simulink model "MAC_ADC"  (R2021a)
settings: Solver=VariableStepAuto  StartTime=0.0  StopTime=1  RelTol=1e-3
values from neighbouring files (symbols this model uses):
  C2 = 2*nb_MAC*minimum_cap    [MAC_ADC_main.m]
  Cf = minimum_cap    [MAC_ADC_main.m]
  clk_freq = 2.1*(nb_cycles_per_sample/(nb_MAC))*sine_frequency_rad    (= 5742.32871594)    [MAC_ADC_main.m]
  clk_period = 1/clk_freq    (= 0.000174145377158)    [MAC_ADC_main.m]
  comparator_high_offset = 0.2*10e-4    (= 0.0002)    [MAC_ADC_main.m]
  comparator_low_offset = -.1*10e-4    (= -0.0001)    [MAC_ADC_main.m]
  comparator_noise_on = non_idealities_on    (= 0)    [MAC_ADC_main.m]
  comparator_noise_rms = 1*k*T* 2/3 / minimum_cap    [MAC_ADC_main.m]
  comparator_offset_on = non_idealities_on    (= 0)    [MAC_ADC_main.m]
  input_BW = 256    [MAC_ADC_main.m]
  k = 1.38064852e-23    [MAC_ADC_main.m]
  leak_current = 2e-15    [MAC_ADC_main.m]
  LNA_bandwidth = 3*input_BW    (= 768)    [MAC_ADC_main.m]
  LNA_gain = 100    [MAC_ADC_main.m]
  LNA_input_referred_noise = min([LNA_input_referred_noise_1,LNA_input_referred_noise_2,LNA_input_referred_noise_3])    [MAC_ADC_main.m]
  LNA_noise_on = non_idealities_on    (= 0)    [MAC_ADC_main.m]
  LNA_SR = I_LNA/(minimum_cap)    [MAC_ADC_main.m]
  MM_attenuation_coeff = C2/(C1+C2)    [MAC_ADC_main.m]
  MM_incomplete_transfer_coeff = C1/(C1+C2)    [MAC_ADC_main.m]
  MM_sampling_noise = ((k*T * C1 / (C1+C2)^2) + (k*T*(C1*C2/(C1+C2))/C2^2))^1/2    [MAC_ADC_main.m]
  nb_cycles_per_sample = number_of_bits + 4 + nb_MAC    (= 34)    [MAC_ADC_main.m]
  nb_MAC = 20    [MAC_ADC_main.m]
  noise_seed = 1    [MAC_ADC_main.m]
  number_of_bits = 10    [MAC_ADC_main.m]
  sampling_gain = Cs/Cf    [MAC_ADC_main.m]
  switch_noise_on = non_idealities_on    (= 0)    [MAC_ADC_main.m]
  switching_noise = k*T/Cf    [MAC_ADC_main.m]
  T = 293    [MAC_ADC_main.m]
  Vref = 2    [MAC_ADC_main.m]
  ZOH_delta = 0*Vref/(2^number_of_bits)    (= 0)    [MAC_ADC_main.m]
libraries: dspsigops x2, simulink x2, simulink_extras x2, spsFirstOrderFilterLib x1, dspsrcs4 x1, dspswit3 x1
settings Model: SnapshotInterval=1  Creator=mac  LastModifiedBy=mac
settings SolverCC: AlgebraicLoopSolver=TrustRegion
settings DataIOCC: SaveFormat=Structure  OutputOption=SpecifiedOutputTimes  OutputTimes=[0:(nb_cycles_per_sample)*clk_period:nb_cycles_per_sample*clk_period*(nb_samples+1)]
settings DebuggingCC: SFMachineParentedDataDiag=warning  UnderSpecifiedDimensionMsg=warning

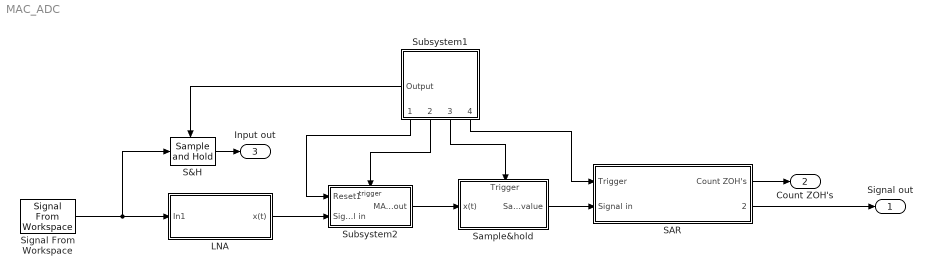
== system MAC_ADC ==
  LNA : Subsystem
      mask Display: text(.5, .5, 'LNA', 'horizontalAlignment', 'center', 'verticalAlignment', 'middle')
  S&H : dspsigops/Sample and Hold  trig=Rising edge  initCond=0  latchinput=off
  SAR : Subsystem
      mask Display: text(.5, .5, 'ZOH SAR', 'horizontalAlignment', 'center', 'verticalAlignment', 'middle')
  Sample&hold : Subsystem
      settings: PortSchema="{\"entries\":[{\"content\":{\"sides\":[{\"content\":{\"connectorIds\":[\"In1\"]},\"type\":\"ConnectorPlacement.EquallySpacedRectSide\",\"uuid\":\"7dc7a4da-613e-4b0b-8b13-7686a16d7398\"},{\"content\":{\"connectorIds\":[\"Out1\"],\"side\":\"RIGHT\"},\"type\":\"ConnectorPlacement.EquallySpacedRectSide\",\"uuid\":\"45e05abc-e512-455b-8082-6639e5b5b38c\"},{\"content\":{\"connectorIds\":[\"In2\"],\"side\":\"TOP\"},\"type\":\"ConnectorPlacement.EquallySpacedRectSide\",\"uuid\":\"b599ec83-17db-48a3-a9e2-86d99bd6436c\"},{\"content\":{\"connectorIds\":[],\"side\":\"HIDDEN\"},\"type\":\"ConnectorPlacement.EquallySpacedRectSide\",\"uuid\":\"38635b0c-9992-4d58-9e3d-95a04571faab\"}]},\"type\":\"ConnectorPlacement.EquallySpacedConnector\",\"uuid\":\"ba0d73a9-648c-4aab-96ad-c6572107f92b\"}],\"packageUris\":[\"http://schema.mathworks.com/mf0/Connector/R2020b\"],\"version\":\"1.0\"}"
      mask Display: text(.5, .5, 'Sample & hold', 'horizontalAlignment', 'center', 'verticalAlignment', 'middle')
  Signal From Workspace : dspsrcs4/Signal From Workspace  X=ADC_input  Ts=1/input_BW  nsamps=1  OutputAfterFinalValue=Setting to zero  ignoreOrWarnInputAndFrameLengths=off  OutputFrames=off
  Subsystem1 : Subsystem
      settings: PortSchema="{\"entries\":[{\"content\":{\"sides\":[{\"content\":{\"connectorIds\":[]},\"type\":\"ConnectorPlacement.EquallySpacedRectSide\",\"uuid\":\"08b362f4-e51c-4c48-9795-383a666f9ced\"},{\"content\":{\"connectorIds\":[\"Out1\",\"Out2\",\"Out3\",\"Out4\"],\"side\":\"RIGHT\"},\"type\":\"ConnectorPlacement.EquallySpacedRectSide\",\"uuid\":\"c1079507-a800-4a5f-bf86-70ea93d83d34\"},{\"content\":{\"connectorIds\":[\"Out5\"],\"side\":\"TOP\"},\"type\":\"ConnectorPlacement.EquallySpacedRectSide\",\"uuid\":\"869febc6-8a73-4083-9381-541b01b45ea7\"},{\"content\":{\"connectorIds\":[],\"side\":\"HIDDEN\"},\"type\":\"ConnectorPlacement.EquallySpacedRectSide\",\"uuid\":\"c096a564-5078-4383-9edd-02cc8c4f8a61\"}]},\"type\":\"ConnectorPlacement.EquallySpacedConnector\",\"uuid\":\"f254d905-503c-4801-8edf-b87de2253b64\"}],\"packageUris\":[\"http://schema.mathworks.com/mf0/Connector/R2020b\"],\"version\":\"1.0\"}"
      mask Display: text(.5, .5, 'Clocking block', 'horizontalAlignment', 'center', 'verticalAlignment', 'middle')
  Subsystem2 : Subsystem
      mask Display: text(.5, .5, 'MAC', 'horizontalAlignment', 'center', 'verticalAlignment', 'middle')
  Signal out : Outport
  Count ZOH's : Outport  Port=2
  Input out : Outport  Port=3
  wires:
  S&H/1 -> Input out/1
  Sample&hold/1(Sampled value) -> SAR/2(Signal in)
  SAR/1(Count ZOH's) -> Count ZOH's/1
  SAR/2(" ") -> Signal out/1
  Subsystem1/4(Output2) -> SAR/1(Trigger)
  Subsystem1/3(Output3) -> Sample&hold/2(Trigger)
  Subsystem1/2(MAC trigger) -> Subsystem2/Trigger
  Subsystem1/1(Output1) -> Subsystem2/1(Reset1)
  Subsystem2/1(MAC_out) -> Sample&hold/1(x(t))
  LNA/1(x(t)) -> Subsystem2/2(Signal in)
  Signal From Workspace/1 -> S&H/1, LNA/1(In1)
  Subsystem1/5(Output) -> S&H/Trigger

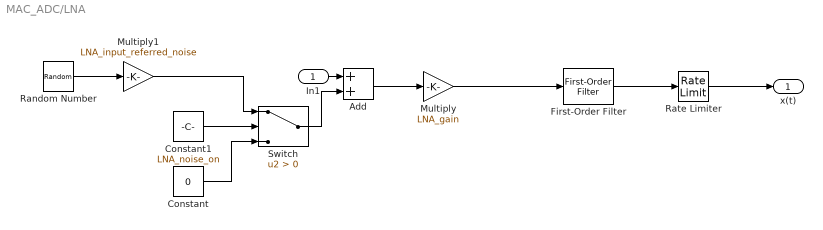
== system MAC_ADC/LNA ==
  In1 : Inport
  Add : Sum
  Constant : Constant  Value=0
  Constant1 : Constant  Value=LNA_noise_on
  First-Order Filter : spsFirstOrderFilterLib/First-Order Filter  FilterType=Lowpass  Tc=1/(LNA_bandwidth*2*pi)  Ts=0  Initialize=off  Vac_Init=[0, 0, 60]  Vdc_Init=0  PlotResponse=off  FreqRange="[0,  200,  1]"
  Multiply : Gain  Gain=LNA_gain
  Multiply1 : Gain  Gain=LNA_input_referred_noise
  Random Number : RandomNumber  Seed=noise_seed+8  SampleTime=clk_period*(number_of_bits+1)
  Rate Limiter : RateLimiter  RisingSlewLimit=LNA_SR  FallingSlewLimit=-LNA_SR  SampleTimeMode=inherited
  Switch : Switch  Criteria=u2 > Threshold
  x(t) : Outport
  wires:
  In1/1 -> Add/1
  Random Number/1 -> Multiply1/1
  Add/1 -> Multiply/1
  Multiply1/1 -> Switch/1
  Constant/1 -> Switch/3
  Constant1/1 -> Switch/2
  Switch/1 -> Add/2
  Multiply/1 -> First-Order Filter/1
  Rate Limiter/1 -> x(t)/1
  First-Order Filter/1 -> Rate Limiter/1

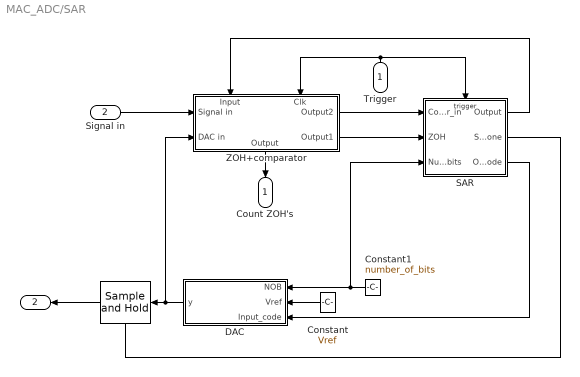
== system MAC_ADC/SAR ==
  Trigger : Inport
  Signal in : Inport  Port=2
  "           " : dspsigops/Sample and Hold  trig=Rising edge  initCond=0  latchinput=off
  Constant : Constant  Value=Vref
  Constant1 : Constant  Value=number_of_bits
  DAC : Subsystem  TreatAsAtomicUnit=on
      mask Display: text(.5, .5, 'DAC', 'horizontalAlignment', 'center', 'verticalAlignment', 'middle')
  SAR : Subsystem  TreatAsAtomicUnit=on
      mask Display: text(.5, .5, 'SAR', 'horizontalAlignment', 'center', 'verticalAlignment', 'middle')
  ZOH+comparator : Subsystem
      settings: PortSchema="{\"entries\":[{\"content\":{\"sides\":[{\"content\":{\"connectorIds\":[\"In1\",\"In2\"]},\"type\":\"ConnectorPlacement.EquallySpacedRectSide\",\"uuid\":\"7512c97b-848f-4506-b4e4-df4323ddef76\"},{\"content\":{\"connectorIds\":[\"Out1\",\"Out2\"],\"side\":\"RIGHT\"},\"type\":\"ConnectorPlacement.EquallySpacedRectSide\",\"uuid\":\"173ab639-376f-4392-8113-9f10a64ef5ba\"},{\"content\":{\"connectorIds\":[\"In3\",\"In4\"],\"side\":\"TOP\"},\"type\":\"ConnectorPlacement.EquallySpacedRectSide\",\"uuid\":\"b167df5d-9d76-4988-887c-42eca149e1c8\"},{\"content\":{\"connectorIds\":[\"Out3\"],\"side\":\"BOTTOM\"},\"type\":\"ConnectorPlacement.EquallySpacedRectSide\",\"uuid\":\"853aabd3-db33-416b-be96-d4661842c69c\"},{\"content\":{\"connectorIds\":[],\"side\":\"HIDDEN\"},\"type\":\"ConnectorPlacement.EquallySpacedRectSide\",\"uuid\":\"e2358589-1082-44c0-a092-f45782973cce\"}]},\"type\":\"ConnectorPlacement.EquallySpacedConnector\",\"uuid\":\"7d04fd09-a295-4450-8277-4727e6a38cb5\"}],\"packageUris\":[\"http://schema.mathworks.com/mf0/Connector/R2020b\"],\"version\":\"1.0\"}"
      mask Display: text(.5, .5, 'Comparator', 'horizontalAlignment', 'center', 'verticalAlignment', 'middle')
  Count ZOH's : Outport
  " " : Outport  Port=2
  wires:
  SAR/2(SAR_done) -> "           "/Trigger
  ZOH+comparator/3(Output) -> Count ZOH's/1
  SAR/3(Output_code) -> DAC/3(Input_code)
  "           "/1 -> " "/1
  Constant/1 -> DAC/2(Vref)
  ZOH+comparator/1(Output2) -> SAR/1(Comparator_in)
  Signal in/1 -> ZOH+comparator/1(Signal in)
  Constant1/1 -> SAR/3(Number of bits), DAC/1(NOB)
  DAC/1(y) -> ZOH+comparator/2(DAC in), "           "/1
  ZOH+comparator/2(Output1) -> SAR/2(ZOH)
  SAR/1(Output) -> ZOH+comparator/3(Input)
  Trigger/1 -> ZOH+comparator/4(Clk), SAR/Trigger

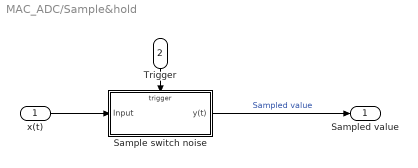
== system MAC_ADC/Sample&hold ==
  x(t) : Inport
  Trigger : Inport  Port=2
  Sample switch noise : Subsystem  TreatAsAtomicUnit=on
  Sampled value : Outport
  wires:
  Trigger/1 -> Sample switch noise/Trigger
  Sample switch noise/1(y(t)) -> Sampled value/1  "Sampled value"
  x(t)/1 -> Sample switch noise/1(Input)

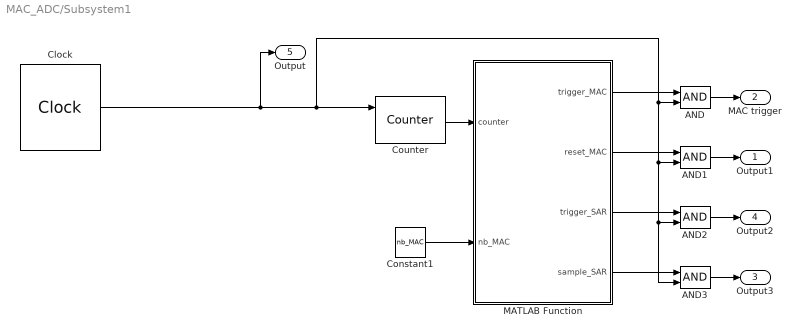
== system MAC_ADC/Subsystem1 ==
  AND{,1..3} (4 alike) : Logic  IconShape=distinctive  AllPortsSameDT=off  OutDataTypeStr=boolean
  Clock : simulink_extras/Flip Flops/Clock  period=clk_period
  Constant1 : Constant  Value=nb_MAC
  Counter : dspswit3/Counter  Direction=Up  CountEvent=Rising edge  CounterSize=User defined  MaxCount=nb_cycles_per_sample-1  InitialCount=0  Output=Count  HitValue=32  ResetInput=on  SamplesPerFrame=1  Ts=1  CntDtype=double  HitDtype=Logical
  MATLAB Function : MATLAB Function  TreatAsAtomicUnit=on
  Output1 : Outport
  MAC trigger : Outport  Port=2
  Output3 : Outport  Port=3
  Output2 : Outport  Port=4
  Output : Outport  Port=5
  wires:
  Clock/1 -> Output/1, Counter/1, AND2/2, AND3/2, AND1/2, AND/2
  Counter/1 -> MATLAB Function/1(counter)
  Constant1/1 -> MATLAB Function/2(nb_MAC)
  AND/1 -> MAC trigger/1
  AND1/1 -> Output1/1
  AND2/1 -> Output2/1
  AND3/1 -> Output3/1
  MATLAB Function/4(sample_SAR) -> AND3/1
  MATLAB Function/3(trigger_SAR) -> AND2/1
  MATLAB Function/2(reset_MAC) -> AND1/1
  MATLAB Function/1(trigger_MAC) -> AND/1

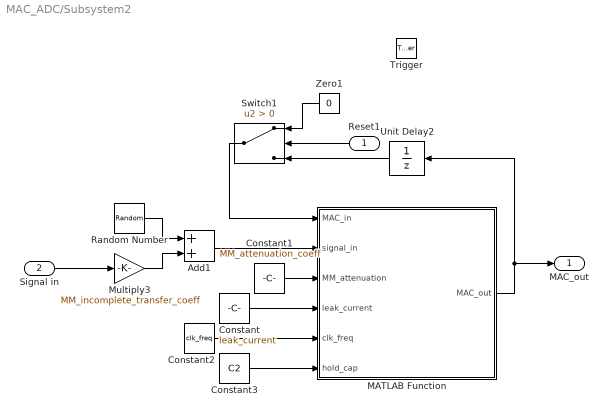
== system MAC_ADC/Subsystem2 ==
  Reset1 : Inport
  Signal in : Inport  Port=2
  Trigger : TriggerPort  VariantControl=Variant  PortDimensions=1
  Add1 : Sum
  Constant : Constant  Value=leak_current
  Constant1 : Constant  Value=MM_attenuation_coeff
  Constant2 : Constant  Value=clk_freq
  Constant3 : Constant  Value=C2
  MATLAB Function : MATLAB Function  TreatAsAtomicUnit=on
  Multiply3 : Gain  Gain=MM_incomplete_transfer_coeff
  Random Number : RandomNumber  Variance=MM_sampling_noise  Seed=noise_seed+2398
  Switch1 : Switch  Criteria=u2 > Threshold
  Unit Delay2 : UnitDelay  InitialCondition=1  SampleTime=-1  HasFrameUpgradeWarning=on
  Zero1 : Constant  Value=0  OutDataTypeStr=Inherit: Inherit via back propagation
  MAC_out : Outport
  wires:
  Zero1/1 -> Switch1/1
  Random Number/1 -> Add1/1
  MATLAB Function/1(MAC_out) -> Unit Delay2/1, MAC_out/1
  Reset1/1 -> Switch1/2
  Constant1/1 -> MATLAB Function/3(MM_attenuation)
  Constant2/1 -> MATLAB Function/5(clk_freq)
  Add1/1 -> MATLAB Function/2(signal_in)
  Signal in/1 -> Multiply3/1
  Multiply3/1 -> Add1/2
  Unit Delay2/1 -> Switch1/3
  Switch1/1 -> MATLAB Function/1(MAC_in)
  Constant/1 -> MATLAB Function/4(leak_current)
  Constant3/1 -> MATLAB Function/6(hold_cap)

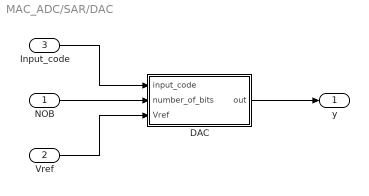
== system MAC_ADC/SAR/DAC ==
  NOB : Inport
  Vref : Inport  Port=2
  Input_code : Inport  Port=3
  DAC : MATLAB Function  TreatAsAtomicUnit=on
  y : Outport
  wires:
  NOB/1 -> DAC/2(number_of_bits)
  Vref/1 -> DAC/3(Vref)
  DAC/1(out) -> y/1
  Input_code/1 -> DAC/1(input_code)

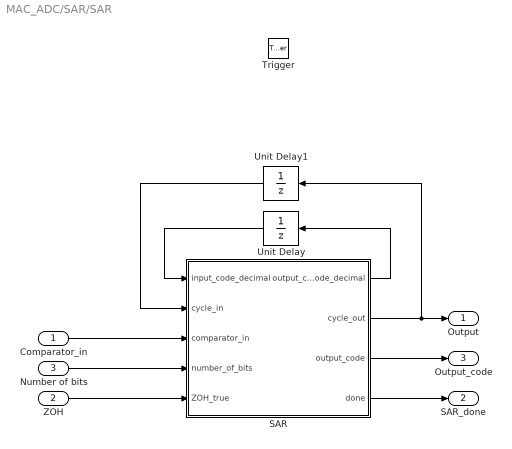
== system MAC_ADC/SAR/SAR ==
  Comparator_in : Inport  LatchByDelayingOutsideSignal=on
  ZOH : Inport  Port=2  LatchByDelayingOutsideSignal=on
  Number of bits : Inport  Port=3
  Trigger : TriggerPort  VariantControl=Variant
  SAR : MATLAB Function  TreatAsAtomicUnit=on
  Unit Delay : UnitDelay  SampleTime=-1  HasFrameUpgradeWarning=on
  Unit Delay1 : UnitDelay  SampleTime=-1  HasFrameUpgradeWarning=on
  Output : Outport
  SAR_done : Outport  Port=2  InitialOutput=0
  Output_code : Outport  Port=3  InitialOutput=zeros(number_of_bits, 1)
      settings: VarSizeSig=Yes
  wires:
  Number of bits/1 -> SAR/4(number_of_bits)
  Comparator_in/1 -> SAR/3(comparator_in)
  Unit Delay1/1 -> SAR/2(cycle_in)
  SAR/3(output_code) -> Output_code/1
  Unit Delay/1 -> SAR/1(input_code_decimal)
  SAR/1(output_code_decimal) -> Unit Delay/1
  SAR/4(done) -> SAR_done/1
  ZOH/1 -> SAR/5(ZOH_true)
  SAR/2(cycle_out) -> Output/1, Unit Delay1/1

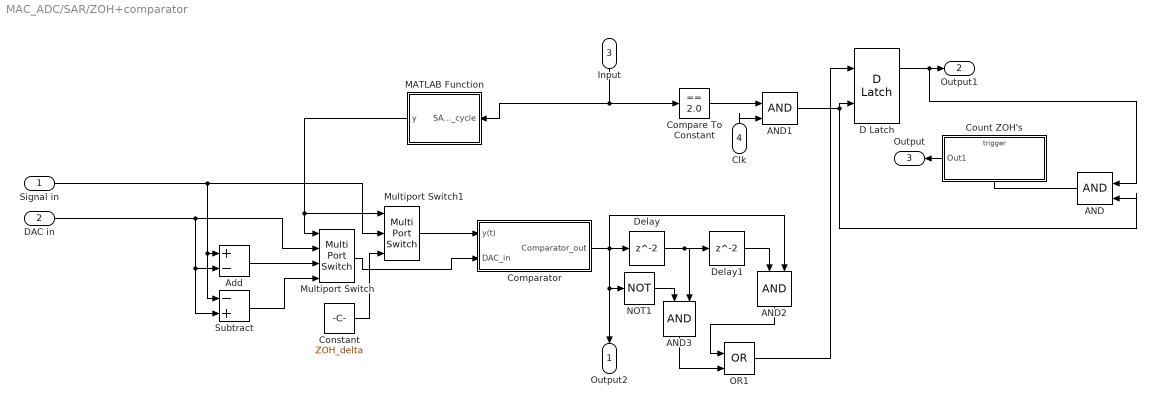
== system MAC_ADC/SAR/ZOH+comparator ==
  Signal in : Inport
  DAC in : Inport  Port=2
  Input : Inport  Port=3
  Clk : Inport  Port=4
  AND{,1..3} (4 alike) : Logic  IconShape=distinctive  AllPortsSameDT=off  OutDataTypeStr=boolean
  Add : Sum  Inputs=+-
  Comparator : Subsystem  TreatAsAtomicUnit=on
      mask Display: text(.5, .5, 'Comparator', 'horizontalAlignment', 'center', 'verticalAlignment', 'middle')
  Compare To Constant : simulink/Logic and Bit Operations/Compare To Constant  relop===  const=2.0  OutDataTypeStr=boolean
  Constant : Constant  Value=ZOH_delta
  Count ZOH's : Subsystem
  D Latch : simulink_extras/Flip Flops/D Latch
      settings: SourceProductBaseCode=SL
  Delay : Delay
  Delay1 : Delay
  MATLAB Function : MATLAB Function  TreatAsAtomicUnit=on
  Multiport Switch : MultiPortSwitch
  Multiport Switch1 : MultiPortSwitch  Inputs=2  DiagnosticForDefault=None
  NOT1 : Logic  Operator=NOT  IconShape=distinctive  AllPortsSameDT=off  OutDataTypeStr=boolean
  OR1 : Logic  Operator=OR  IconShape=distinctive  AllPortsSameDT=off  OutDataTypeStr=boolean
  Subtract : Sum  Inputs=-+
  Output2 : Outport
  Output1 : Outport  Port=2
  Output : Outport  Port=3
  wires:
  Delay/1 -> Delay1/1, AND3/2
  Constant/1 -> Multiport Switch1/3
  DAC in/1 -> Multiport Switch/2, Subtract/2, Add/2
  D Latch/1 -> AND/1, Output1/1
  Add/1 -> Multiport Switch/3
  Signal in/1 -> Subtract/1, Add/1, Multiport Switch1/2
  Multiport Switch1/1 -> Comparator/1(y(t))
  Comparator/1(Comparator_out) -> Delay/1, AND2/2, Output2/1, NOT1/1
  Delay1/1 -> AND2/1
  MATLAB Function/1(y) -> Multiport Switch1/1, Multiport Switch/1
  Input/1 -> Compare To Constant/1, MATLAB Function/1(SAR_clk_cycle)
  Compare To Constant/1 -> AND1/1
  Count ZOH's/1(Out1) -> Output/1
  Multiport Switch/1 -> Comparator/2(DAC_in)
  OR1/1 -> D Latch/1
  Subtract/1 -> Multiport Switch/4
  NOT1/1 -> AND3/1
  AND3/1 -> OR1/2
  AND2/1 -> OR1/1
  AND/1 -> Count ZOH's/Trigger
  Clk/1 -> AND1/2
  AND1/1 -> D Latch/2, AND/2

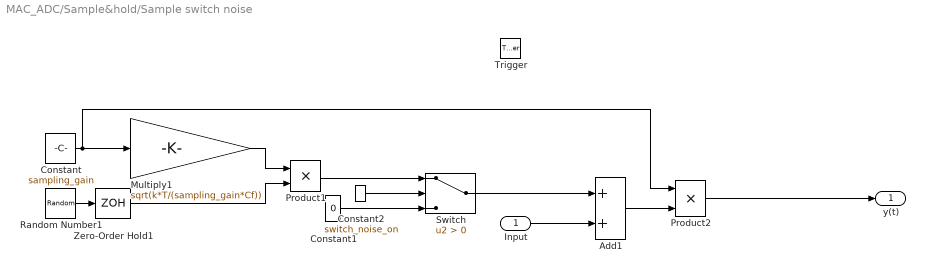
== system MAC_ADC/Sample&hold/Sample switch noise ==
  Input : Inport
  Trigger : TriggerPort  VariantControl=Variant
  Add1 : Sum
  Constant : Constant  Value=sampling_gain
  Constant1 : Constant  Value=0
  Constant2 : Constant  Value=switch_noise_on
  Multiply1 : Gain  Gain=sqrt(k*T/(sampling_gain*Cf))  OutDataTypeStr=Inherit: Same as input
  Product1 : Product
  Product2 : Product
  Random Number1 : RandomNumber  Variance=switching_noise  Seed=noise_seed+2
  Switch : Switch  Criteria=u2 > Threshold
  Zero-Order Hold1 : ZeroOrderHold  SampleTime=-1
  y(t) : Outport
  wires:
  Product2/1 -> y(t)/1
  Random Number1/1 -> Zero-Order Hold1/1
  Multiply1/1 -> Product1/1
  Add1/1 -> Product2/2
  Constant/1 -> Product2/1, Multiply1/1
  Constant2/1 -> Switch/2
  Constant1/1 -> Switch/3
  Product1/1 -> Switch/1
  Zero-Order Hold1/1 -> Product1/2
  Switch/1 -> Add1/1
  Input/1 -> Add1/2

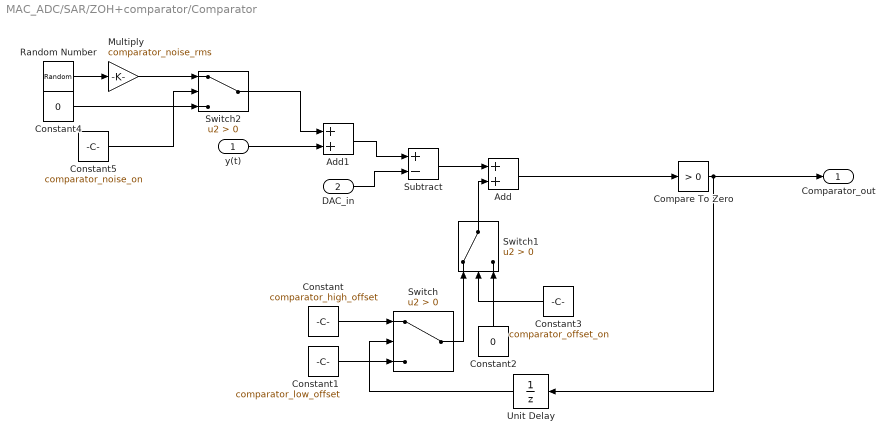
== system MAC_ADC/SAR/ZOH+comparator/Comparator ==
  y(t) : Inport
  DAC_in : Inport  Port=2
  Add : Sum
  Add1 : Sum
  Compare To Zero : simulink/Logic and Bit Operations/Compare To Zero  relop=>  OutDataTypeStr=boolean
  Constant : Constant  Value=comparator_high_offset
  Constant1 : Constant  Value=comparator_low_offset
  Constant2 : Constant  Value=0
  Constant3 : Constant  Value=comparator_offset_on
  Constant4 : Constant  Value=0
  Constant5 : Constant  Value=comparator_noise_on
  Multiply : Gain  Gain=comparator_noise_rms
  Random Number : RandomNumber  SampleTime=1/clk_freq
  Subtract : Sum  Inputs=+-
  Switch : Switch  Criteria=u2 > Threshold
  Switch1 : Switch  Criteria=u2 > Threshold
  Switch2 : Switch  Criteria=u2 > Threshold
  Unit Delay : UnitDelay  SampleTime=-1  HasFrameUpgradeWarning=on
  Comparator_out : Outport
  wires:
  Switch/1 -> Switch1/1
  Subtract/1 -> Add/1
  Constant/1 -> Switch/1
  Constant2/1 -> Switch1/3
  Add/1 -> Compare To Zero/1
  Switch1/1 -> Add/2
  Constant3/1 -> Switch1/2
  Unit Delay/1 -> Switch/2
  Constant1/1 -> Switch/3
  DAC_in/1 -> Subtract/2
  Add1/1 -> Subtract/1
  y(t)/1 -> Add1/2
  Random Number/1 -> Multiply/1
  Switch2/1 -> Add1/1
  Multiply/1 -> Switch2/1
  Constant4/1 -> Switch2/3
  Constant5/1 -> Switch2/2
  Compare To Zero/1 -> Unit Delay/1, Comparator_out/1

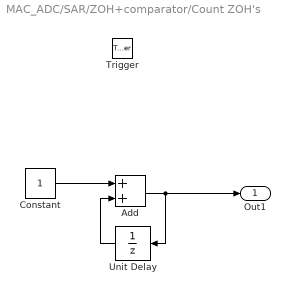
== system MAC_ADC/SAR/ZOH+comparator/Count ZOH's ==
  Trigger : TriggerPort  VariantControl=Variant  PortDimensions=1
  Add : Sum  AccumDataTypeStr=double  OutDataTypeStr=double
  Constant : Constant
  Unit Delay : UnitDelay  SampleTime=-1  HasFrameUpgradeWarning=on
  Out1 : Outport
  wires:
  Constant/1 -> Add/1
  Add/1 -> Unit Delay/1, Out1/1
  Unit Delay/1 -> Add/2

== matlab function MAC_ADC/SAR/ZOH+comparator/MATLAB Function ==
  data: SAR_clk_cycle input; y output
function y = fcn(SAR_clk_cycle)
    if (SAR_clk_cycle)==0
        y = 2;
    elseif (SAR_clk_cycle)==1
        y=3;
    else
        y=1;
    end
end

== matlab function MAC_ADC/SAR/DAC/DAC ==
  data: input_code input size=number_of_bits; out output double size=1; number_of_bits input; Vref input
function out = fcn(input_code, number_of_bits, Vref)
out = Vref/(2^number_of_bits) * (bi2de(input_code.', 'left-msb'));
end

== matlab function MAC_ADC/SAR/SAR/SAR ==
  data: output_code_decimal output size=1; cycle_out output size=1; output_code output size=number_of_bits; input_code_decimal input; cycle_in input; comparator_in input; number_of_bits input; done output; ZOH_true input
function [output_code_decimal, cycle_out, output_code, done] = fcn(input_code_decimal, cycle_in, comparator_in, number_of_bits, ZOH_true)

    input_code = de2bi(input_code_decimal, 'left-msb');
    output_code = [zeros(number_of_bits-size(input_code.',1),1); input_code.'];
    cycle_out = cycle_in + 1;
    done = 0;

    if (cycle_in < 2)
        
        % Wait for ZOH to be determined
        
    elseif (cycle_in == 2)
        % Reset output code, start SA algorithm unless ZOH
        if (~ZOH_true)
            output_code = zeros(number_of_bits,1);
            output_code(1, 1) = 1;
        end
        
    elseif (cycle_in == number_of_bits+2)
        % Finish SA algorithm unless ZOH, set done & reset output_cycle
        done = 1;
        if (~ZOH_true)
            output_code(number_of_bits,1) = comparator_in;
        end
        cycle_out = 0;
    else
        % Continue SA algorithm unless ZOH
        if (~ZOH_true)
            if (comparator_in == 0)
                output_code(cycle_in-2,1) = 0;
            end

            output_code(cycle_in-1,1) = 1;
        end
        
    end
    
    output_code_decimal_temp = bi2de(output_code.', 'left-msb');
    output_code_decimal = output_code_decimal_temp(1,1);
end

== matlab function MAC_ADC/Subsystem1/MATLAB Function ==
  data: counter input; trigger_MAC output; nb_MAC input; reset_MAC output; trigger_SAR output; sample_SAR output
function [trigger_MAC, reset_MAC, trigger_SAR, sample_SAR] = control_logic(counter, nb_MAC)

    trigger_MAC = 0;
    reset_MAC = 0;
    trigger_SAR = 0;
    sample_SAR = 0;

    if (counter <= nb_MAC-1) 
        trigger_MAC = 1;
        
        if (counter == 0)
            reset_MAC = 1;
        end
        
    elseif (counter == nb_MAC)
        sample_SAR = 1;
        
    else
        trigger_SAR = 1;
    end
end

== matlab function MAC_ADC/Subsystem2/MATLAB Function ==
  data: MAC_in input; signal_in input; MAC_out output; MM_attenuation input; leak_current input; clk_freq input; hold_cap input
function MAC_out = fcn(MAC_in, signal_in, MM_attenuation, leak_current, clk_freq, hold_cap)

MAC_out = signal_in + MM_attenuation*MAC_in;
MAC_out = max(0,MAC_out - leak_current/(clk_freq*hold_cap));

end
